simulink library "cdsSWD"  (Simulink 6.2)
settings Model: LastModifiedBy=rolf

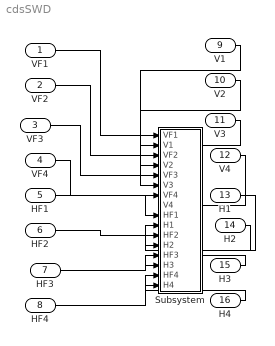
== system cdsSWD ==
  VF1 : Inport  Port=1  LatchInput=off
  VF2 : Inport  Port=2  LatchInput=off
  VF3 : Inport  Port=3  LatchInput=off
  VF4 : Inport  Port=4  LatchInput=off
  HF1 : Inport  Port=5  LatchInput=off
  HF2 : Inport  Port=6  LatchInput=off
  HF3 : Inport  Port=7  LatchInput=off
  HF4 : Inport  Port=8  LatchInput=off
  V1 : Inport  Port=9  LatchInput=off
  V2 : Inport  Port=10  LatchInput=off
  V3 : Inport  Port=11  LatchInput=off
  V4 : Inport  Port=12  LatchInput=off
  H1 : Inport  Port=13  LatchInput=off
  H2 : Inport  Port=14  LatchInput=off
  H3 : Inport  Port=15  LatchInput=off
  H4 : Inport  Port=16  LatchInput=off
  Subsystem : Subsystem
  wires:
  VF1/1 -> Subsystem/1(VF1)
  VF2/1 -> Subsystem/3(VF2)
  VF3/1 -> Subsystem/5(VF3)
  VF4/1 -> Subsystem/7(VF4)
  HF1/1 -> Subsystem/9(HF1)
  HF2/1 -> Subsystem/11(HF2)
  HF3/1 -> Subsystem/13(HF3)
  HF4/1 -> Subsystem/15(HF4)
  V1/1 -> Subsystem/2(V1)
  V2/1 -> Subsystem/4(V2)
  V3/1 -> Subsystem/6(V3)
  V4/1 -> Subsystem/8(V4)
  H1/1 -> Subsystem/10(H1)
  H2/1 -> Subsystem/12(H2)
  H3/1 -> Subsystem/14(H3)
  H4/1 -> Subsystem/16(H4)

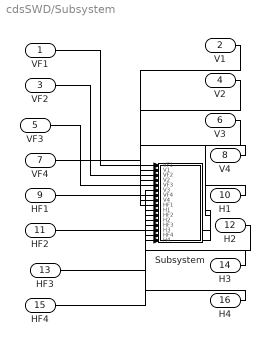
== system cdsSWD/Subsystem ==
  VF1 : Inport  Port=1  LatchInput=off
  V1 : Inport  Port=2  LatchInput=off
  VF2 : Inport  Port=3  LatchInput=off
  V2 : Inport  Port=4  LatchInput=off
  VF3 : Inport  Port=5  LatchInput=off
  V3 : Inport  Port=6  LatchInput=off
  VF4 : Inport  Port=7  LatchInput=off
  V4 : Inport  Port=8  LatchInput=off
  HF1 : Inport  Port=9  LatchInput=off
  H1 : Inport  Port=10  LatchInput=off
  HF2 : Inport  Port=11  LatchInput=off
  H2 : Inport  Port=12  LatchInput=off
  HF3 : Inport  Port=13  LatchInput=off
  H3 : Inport  Port=14  LatchInput=off
  HF4 : Inport  Port=15  LatchInput=off
  H4 : Inport  Port=16  LatchInput=off
  Subsystem : Subsystem
  wires:
  VF1/1 -> Subsystem/1(VF1)
  V1/1 -> Subsystem/2(V1)
  VF2/1 -> Subsystem/3(VF2)
  V2/1 -> Subsystem/4(V2)
  VF3/1 -> Subsystem/5(VF3)
  V3/1 -> Subsystem/6(V3)
  VF4/1 -> Subsystem/7(VF4)
  V4/1 -> Subsystem/8(V4)
  HF1/1 -> Subsystem/9(HF1)
  H1/1 -> Subsystem/10(H1)
  HF2/1 -> Subsystem/11(HF2)
  H2/1 -> Subsystem/12(H2)
  HF3/1 -> Subsystem/13(HF3)
  H3/1 -> Subsystem/14(H3)
  HF4/1 -> Subsystem/15(HF4)
  H4/1 -> Subsystem/16(H4)

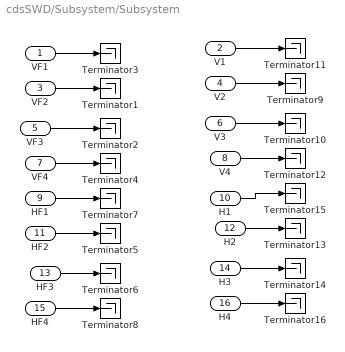
== system cdsSWD/Subsystem/Subsystem ==
  VF1 : Inport  Port=1  LatchInput=off
  V1 : Inport  Port=2  LatchInput=off
  VF2 : Inport  Port=3  LatchInput=off
  V2 : Inport  Port=4  LatchInput=off
  VF3 : Inport  Port=5  LatchInput=off
  V3 : Inport  Port=6  LatchInput=off
  VF4 : Inport  Port=7  LatchInput=off
  V4 : Inport  Port=8  LatchInput=off
  HF1 : Inport  Port=9  LatchInput=off
  H1 : Inport  Port=10  LatchInput=off
  HF2 : Inport  Port=11  LatchInput=off
  H2 : Inport  Port=12  LatchInput=off
  HF3 : Inport  Port=13  LatchInput=off
  H3 : Inport  Port=14  LatchInput=off
  HF4 : Inport  Port=15  LatchInput=off
  H4 : Inport  Port=16  LatchInput=off
  Terminator{1..16} (16 alike) : Terminator
  wires:
  V1/1 -> Terminator11/1
  V2/1 -> Terminator9/1
  V3/1 -> Terminator10/1
  V4/1 -> Terminator12/1
  H1/1 -> Terminator15/1
  H2/1 -> Terminator13/1
  H3/1 -> Terminator14/1
  H4/1 -> Terminator16/1
  VF1/1 -> Terminator3/1
  VF2/1 -> Terminator1/1
  VF3/1 -> Terminator2/1
  VF4/1 -> Terminator4/1
  HF1/1 -> Terminator7/1
  HF2/1 -> Terminator5/1
  HF3/1 -> Terminator6/1
  HF4/1 -> Terminator8/1
